simulink model "AirCtl_CtlValCalc"  (R2016b)
settings: configuration reference "CodeGenConfigSet" (kept outside this file)
values from neighbouring files (symbols this model uses):
  AirCtl_drCtlValDec_CUR = Calibration.Parameter    [init_AirCtl_CtlValCalc.m]    (also in init_AirCtl_CtlValCalc_SIL.m = Simulink.Parameter)
  AirCtl_drCtlValDec_CURX = Calibration.Parameter    [init_AirCtl_CtlValCalc.m]    (also in init_AirCtl_CtlValCalc_SIL.m = Simulink.Parameter)
  AirCtl_drCtlValDwn_C = Calibration.Parameter    [init_AirCtl_CtlValCalc.m]    (also in init_AirCtl_CtlValCalc_SIL.m = Simulink.Parameter)
  AirCtl_drCtlValInc_CUR = Calibration.Parameter    [init_AirCtl_CtlValCalc.m]    (also in init_AirCtl_CtlValCalc_SIL.m = Simulink.Parameter)
  AirCtl_drCtlValInc_CURX = Calibration.Parameter    [init_AirCtl_CtlValCalc.m]    (also in init_AirCtl_CtlValCalc_SIL.m = Simulink.Parameter)
  AirCtl_drCtlValUp_C = Calibration.Parameter    [init_AirCtl_CtlValCalc.m]    (also in init_AirCtl_CtlValCalc_SIL.m = Simulink.Parameter)
  AirCtl_facCtlAirTempCorEOM0_CUR = Calibration.Parameter    [init_AirCtl_CtlValCalc.m]    (also in init_AirCtl_CtlValCalc_SIL.m = Simulink.Parameter)
  AirCtl_facCtlAirTempCorEOM0_CURX = Calibration.Parameter    [init_AirCtl_CtlValCalc.m]    (also in init_AirCtl_CtlValCalc_SIL.m = Simulink.Parameter)
  AirCtl_facCtlEngTempCorEOM0_CUR = Calibration.Parameter    [init_AirCtl_CtlValCalc.m]    (also in init_AirCtl_CtlValCalc_SIL.m = Simulink.Parameter)
  AirCtl_facCtlEngTempCorEOM0_CURX = Calibration.Parameter    [init_AirCtl_CtlValCalc.m]    (also in init_AirCtl_CtlValCalc_SIL.m = Simulink.Parameter)
  AirCtl_facEngTempSmkDynCor_CUR = Calibration.Parameter    [init_AirCtl_CtlValCalc.m]    (also in init_AirCtl_CtlValCalc_SIL.m = Simulink.Parameter)
  AirCtl_facEngTempSmkDynCor_CURX = Calibration.Parameter    [init_AirCtl_CtlValCalc.m]    (also in init_AirCtl_CtlValCalc_SIL.m = Simulink.Parameter)
  AirCtl_facEngTempSmkStatCor_CUR = Calibration.Parameter    [init_AirCtl_CtlValCalc.m]    (also in init_AirCtl_CtlValCalc_SIL.m = Simulink.Parameter)
  AirCtl_facEngTempSmkStatCor_CURX = Calibration.Parameter    [init_AirCtl_CtlValCalc.m]    (also in init_AirCtl_CtlValCalc_SIL.m = Simulink.Parameter)
  AirCtl_facEnvPresCtlVal_CUR = Calibration.Parameter    [init_AirCtl_CtlValCalc.m]    (also in init_AirCtl_CtlValCalc_SIL.m = Simulink.Parameter)
  AirCtl_facEnvPresCtlVal_CURX = Calibration.Parameter    [init_AirCtl_CtlValCalc.m]    (also in init_AirCtl_CtlValCalc_SIL.m = Simulink.Parameter)
  AirCtl_facWrmUpCtlVal_CUR = Calibration.Parameter    [init_AirCtl_CtlValCalc.m]    (also in init_AirCtl_CtlValCalc_SIL.m = Simulink.Parameter)
  AirCtl_facWrmUpCtlVal_CURX = Calibration.Parameter    [init_AirCtl_CtlValCalc.m]    (also in init_AirCtl_CtlValCalc_SIL.m = Simulink.Parameter)
  AirCtl_numAirTempCtlVal_C = Calibration.Parameter    [init_AirCtl_CtlValCalc.m]    (also in init_AirCtl_CtlValCalc_SIL.m = Simulink.Parameter)
  AirCtl_numEngTempCtlVal_C = Calibration.Parameter    [init_AirCtl_CtlValCalc.m]    (also in init_AirCtl_CtlValCalc_SIL.m = Simulink.Parameter)
  AirCtl_rCtlAirTempCorEOM0_MAP = Calibration.Parameter    [init_AirCtl_CtlValCalc.m]    (also in init_AirCtl_CtlValCalc_SIL.m = Simulink.Parameter)
  AirCtl_rCtlAirTempCorEOM0_MAPX = Calibration.Parameter    [init_AirCtl_CtlValCalc.m]    (also in init_AirCtl_CtlValCalc_SIL.m = Simulink.Parameter)
  AirCtl_rCtlAirTempCorEOM0_MAPY = Calibration.Parameter    [init_AirCtl_CtlValCalc.m]    (also in init_AirCtl_CtlValCalc_SIL.m = Simulink.Parameter)
  AirCtl_rCtlCorBasEOM0_MAP = Calibration.Parameter    [init_AirCtl_CtlValCalc.m]    (also in init_AirCtl_CtlValCalc_SIL.m = Simulink.Parameter)
  AirCtl_rCtlCorBasEOM0_MAPX = Calibration.Parameter    [init_AirCtl_CtlValCalc.m]    (also in init_AirCtl_CtlValCalc_SIL.m = Simulink.Parameter)
  AirCtl_rCtlCorBasEOM0_MAPY = Calibration.Parameter    [init_AirCtl_CtlValCalc.m]    (also in init_AirCtl_CtlValCalc_SIL.m = Simulink.Parameter)
  AirCtl_rCtlEngTempCorEOM0_MAP = Calibration.Parameter    [init_AirCtl_CtlValCalc.m]    (also in init_AirCtl_CtlValCalc_SIL.m = Simulink.Parameter)
  AirCtl_rCtlEngTempCorEOM0_MAPX = Calibration.Parameter    [init_AirCtl_CtlValCalc.m]    (also in init_AirCtl_CtlValCalc_SIL.m = Simulink.Parameter)
  AirCtl_rCtlEngTempCorEOM0_MAPY = Calibration.Parameter    [init_AirCtl_CtlValCalc.m]    (also in init_AirCtl_CtlValCalc_SIL.m = Simulink.Parameter)
  AirCtl_rCtlEnvPresCorEOM0_MAP = Calibration.Parameter    [init_AirCtl_CtlValCalc.m]    (also in init_AirCtl_CtlValCalc_SIL.m = Simulink.Parameter)
  AirCtl_rCtlEnvPresCorEOM0_MAPX = Calibration.Parameter    [init_AirCtl_CtlValCalc.m]    (also in init_AirCtl_CtlValCalc_SIL.m = Simulink.Parameter)
  AirCtl_rCtlEnvPresCorEOM0_MAPY = Calibration.Parameter    [init_AirCtl_CtlValCalc.m]    (also in init_AirCtl_CtlValCalc_SIL.m = Simulink.Parameter)
  AirCtl_rCtlValBasEOM0_MAP = Calibration.Parameter    [init_AirCtl_CtlValCalc.m]    (also in init_AirCtl_CtlValCalc_SIL.m = Simulink.Parameter)
  AirCtl_rCtlValBasEOM0_MAPX = Calibration.Parameter    [init_AirCtl_CtlValCalc.m]    (also in init_AirCtl_CtlValCalc_SIL.m = Simulink.Parameter)
  AirCtl_rCtlValBasEOM0_MAPY = Calibration.Parameter    [init_AirCtl_CtlValCalc.m]    (also in init_AirCtl_CtlValCalc_SIL.m = Simulink.Parameter)
  AirCtl_rEngTempSmkDynCor_MAP = Calibration.Parameter    [init_AirCtl_CtlValCalc.m]    (also in init_AirCtl_CtlValCalc_SIL.m = Simulink.Parameter)
  AirCtl_rEngTempSmkDynCor_MAPX = Calibration.Parameter    [init_AirCtl_CtlValCalc.m]    (also in init_AirCtl_CtlValCalc_SIL.m = Simulink.Parameter)
  AirCtl_rEngTempSmkDynCor_MAPY = Calibration.Parameter    [init_AirCtl_CtlValCalc.m]    (also in init_AirCtl_CtlValCalc_SIL.m = Simulink.Parameter)
  AirCtl_rEngTempSmkStatCor_MAP = Calibration.Parameter    [init_AirCtl_CtlValCalc.m]    (also in init_AirCtl_CtlValCalc_SIL.m = Simulink.Parameter)
  AirCtl_rEngTempSmkStatCor_MAPX = Calibration.Parameter    [init_AirCtl_CtlValCalc.m]    (also in init_AirCtl_CtlValCalc_SIL.m = Simulink.Parameter)
  AirCtl_rEngTempSmkStatCor_MAPY = Calibration.Parameter    [init_AirCtl_CtlValCalc.m]    (also in init_AirCtl_CtlValCalc_SIL.m = Simulink.Parameter)
  AirCtl_rEnvPresCtlVal_MAP = Calibration.Parameter    [init_AirCtl_CtlValCalc.m]    (also in init_AirCtl_CtlValCalc_SIL.m = Simulink.Parameter)
  AirCtl_rEnvPresCtlVal_MAPX = Calibration.Parameter    [init_AirCtl_CtlValCalc.m]    (also in init_AirCtl_CtlValCalc_SIL.m = Simulink.Parameter)
  AirCtl_rEnvPresCtlVal_MAPY = Calibration.Parameter    [init_AirCtl_CtlValCalc.m]    (also in init_AirCtl_CtlValCalc_SIL.m = Simulink.Parameter)
  AirCtl_rSmkDyn_MAP = Calibration.Parameter    [init_AirCtl_CtlValCalc.m]    (also in init_AirCtl_CtlValCalc_SIL.m = Simulink.Parameter)
  AirCtl_rSmkDyn_MAPX = Calibration.Parameter    [init_AirCtl_CtlValCalc.m]    (also in init_AirCtl_CtlValCalc_SIL.m = Simulink.Parameter)
  AirCtl_rSmkDyn_MAPY = Calibration.Parameter    [init_AirCtl_CtlValCalc.m]    (also in init_AirCtl_CtlValCalc_SIL.m = Simulink.Parameter)
  AirCtl_rSmkStat_MAP = Calibration.Parameter    [init_AirCtl_CtlValCalc.m]    (also in init_AirCtl_CtlValCalc_SIL.m = Simulink.Parameter)
  AirCtl_rSmkStat_MAPX = Calibration.Parameter    [init_AirCtl_CtlValCalc.m]    (also in init_AirCtl_CtlValCalc_SIL.m = Simulink.Parameter)
  AirCtl_rSmkStat_MAPY = Calibration.Parameter    [init_AirCtl_CtlValCalc.m]    (also in init_AirCtl_CtlValCalc_SIL.m = Simulink.Parameter)
  AirCtl_rWrmUpCtlVal_MAP = Calibration.Parameter    [init_AirCtl_CtlValCalc.m]    (also in init_AirCtl_CtlValCalc_SIL.m = Simulink.Parameter)
  AirCtl_rWrmUpCtlVal_MAPX = Calibration.Parameter    [init_AirCtl_CtlValCalc.m]    (also in init_AirCtl_CtlValCalc_SIL.m = Simulink.Parameter)
  AirCtl_rWrmUpCtlVal_MAPY = Calibration.Parameter    [init_AirCtl_CtlValCalc.m]    (also in init_AirCtl_CtlValCalc_SIL.m = Simulink.Parameter)
  AirCtl_swtAirMs_C = Calibration.Parameter    [init_AirCtl_CtlValCalc.m]    (also in init_AirCtl_CtlValCalc_SIL.m = Simulink.Parameter)
undefined symbols (not defined in the file or in its folder): AirCtl_CtlValCalc_DT, Switch_conv
libraries: CXLib x6
settings Model: Creator=lvzhanghui  LastModifiedBy=zhulinfeng
settings ConfigSetRef: SourceLocation=Base Workspace

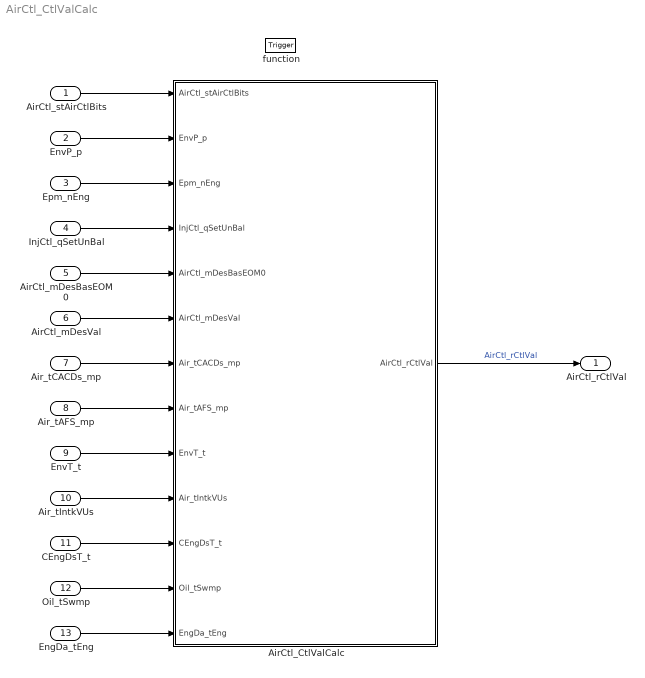
== system AirCtl_CtlValCalc ==
  AirCtl_stAirCtlBits : Inport  Description=Status of the switch-off events of the exhaust-gas recirculation control, monitoring  OutMin=0  OutMax=4294967295  OutDataTypeStr=State_uint32
  EnvP_p : Inport  Tag=kPa  Description=Barometric pressure  Port=2  OutMin=0  OutMax=3276  OutDataTypeStr=AirPressure_kPa
  Epm_nEng : Inport  Tag=rpm  Description=Engine speed  Port=3  OutMin=0  OutMax=6000  OutDataTypeStr=EngSpeed_rpm
  InjCtl_qSetUnBal : Inport  Tag=mg/hub  Description=Current injection quantity  Port=4  OutMin=-319  OutMax=319  OutDataTypeStr=FuelMass_mg_hub
  AirCtl_mDesBasEOM0 : Inport  Tag=mg/hub  Description=Base air mass setpoint value from the basic map  Port=5  OutMin=-15000  OutMax=15000  OutDataTypeStr=AirMass_mg_hub
  AirCtl_mDesVal : Inport  Tag=mg/hub  Description=Desired air mass  Port=6  OutMin=-15000  OutMax=15000  OutDataTypeStr=AirMass_mg_hub
  Air_tCACDs_mp : Inport  Tag=deg  Description=Charge-air temperature downstream from charge-air cooler  Port=7  OutMin=-200  OutMax=200  OutDataTypeStr=Temp_deg
  Air_tAFS_mp : Inport  Tag=deg  Description=Induction air temperature at the HFM  Port=8  OutMin=-200  OutMax=200  OutDataTypeStr=Temp_deg
  EnvT_t : Inport  Tag=deg  Description=Environmental temperature  Port=9  OutMin=-200  OutMax=200  OutDataTypeStr=Temp_deg
  Air_tIntkVUs : Inport  Tag=deg  Description=Intake air temperature upstream of the inlet valve  Port=10  OutMin=-200  OutMax=200  OutDataTypeStr=Temp_deg
  CEngDsT_t : Inport  Tag=deg  Description=engine coolant temperature after filter  Port=11  OutMin=-200  OutMax=200  OutDataTypeStr=Temp_deg
  Oil_tSwmp : Inport  Tag=deg  Description=Oil temperature in oil sump  Port=12  OutMin=-50  OutMax=200  OutDataTypeStr=Temp_deg
  EngDa_tEng : Inport  Tag=deg  Description=Engine temperature  Port=13  OutMin=-1000  OutMax=1000  OutDataTypeStr=Temp_deg
  function : TriggerPort  TriggerType=function-call  VariantControl=Variant
  AirCtl_CtlValCalc : Subsystem
  AirCtl_rCtlVal : Outport  Tag=%  Description=Stationary part of controlled variable  OutMin=-100  OutMax=100  OutDataTypeStr=Prc_100_rate
  wires:
  AirCtl_CtlValCalc/1(AirCtl_rCtlVal) -> AirCtl_rCtlVal/1  "AirCtl_rCtlVal"
  EngDa_tEng/1 -> AirCtl_CtlValCalc/13(EngDa_tEng)
  Oil_tSwmp/1 -> AirCtl_CtlValCalc/12(Oil_tSwmp)
  CEngDsT_t/1 -> AirCtl_CtlValCalc/11(CEngDsT_t)
  Air_tIntkVUs/1 -> AirCtl_CtlValCalc/10(Air_tIntkVUs)
  EnvT_t/1 -> AirCtl_CtlValCalc/9(EnvT_t)
  Air_tAFS_mp/1 -> AirCtl_CtlValCalc/8(Air_tAFS_mp)
  Air_tCACDs_mp/1 -> AirCtl_CtlValCalc/7(Air_tCACDs_mp)
  AirCtl_mDesVal/1 -> AirCtl_CtlValCalc/6(AirCtl_mDesVal)
  AirCtl_mDesBasEOM0/1 -> AirCtl_CtlValCalc/5(AirCtl_mDesBasEOM0)
  InjCtl_qSetUnBal/1 -> AirCtl_CtlValCalc/4(InjCtl_qSetUnBal)
  Epm_nEng/1 -> AirCtl_CtlValCalc/3(Epm_nEng)
  EnvP_p/1 -> AirCtl_CtlValCalc/2(EnvP_p)
  AirCtl_stAirCtlBits/1 -> AirCtl_CtlValCalc/1(AirCtl_stAirCtlBits)

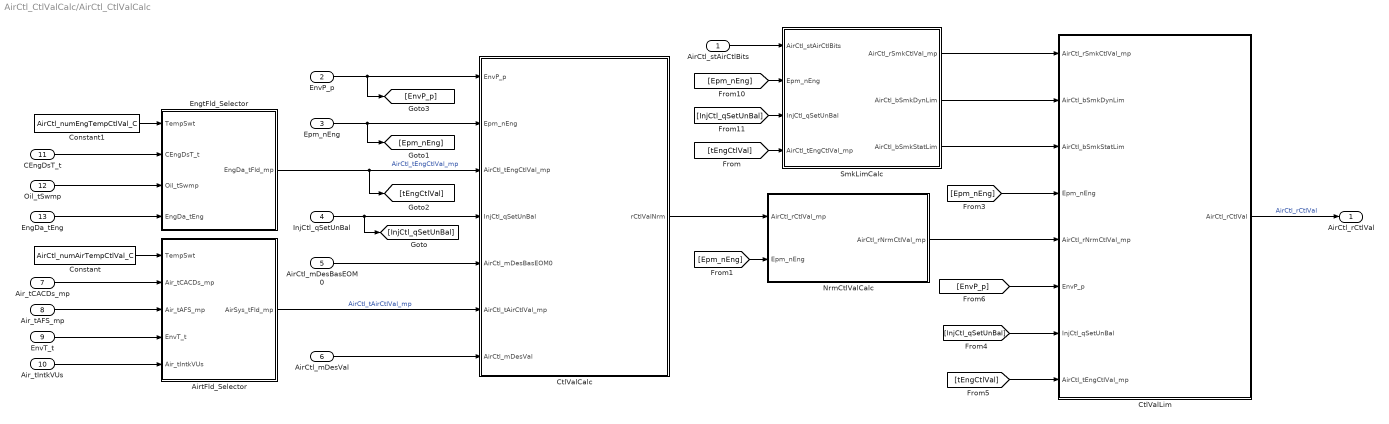
== system AirCtl_CtlValCalc/AirCtl_CtlValCalc ==
  AirCtl_stAirCtlBits : Inport
  EnvP_p : Inport  Tag=kPa  Port=2
  Epm_nEng : Inport  Tag=rpm  Port=3
  InjCtl_qSetUnBal : Inport  Tag=mg/hub  Port=4
  AirCtl_mDesBasEOM0 : Inport  Tag=mg/hub  Port=5
  AirCtl_mDesVal : Inport  Tag=mg/hub  Port=6
  Air_tCACDs_mp : Inport  Tag=deg  Port=7
  Air_tAFS_mp : Inport  Tag=deg  Port=8
  EnvT_t : Inport  Tag=deg  Port=9
  Air_tIntkVUs : Inport  Tag=deg  Port=10
  CEngDsT_t : Inport  Tag=deg  Port=11
  Oil_tSwmp : Inport  Tag=deg  Port=12
  EngDa_tEng : Inport  Tag=deg  Port=13
  AirtFld_Selector : Subsystem
  Constant : Constant  Value=AirCtl_numAirTempCtlVal_C
  Constant1 : Constant  Value=AirCtl_numEngTempCtlVal_C
  CtlValCalc : Subsystem
  CtlValLim : Subsystem
  EngtFld_Selector : Subsystem
  NrmCtlValCalc : Subsystem
  SmkLimCalc : Subsystem
  AirCtl_rCtlVal : Outport  Tag=%
  wires:
  SmkLimCalc/2(AirCtl_bSmkDynLim) -> CtlValLim/2(AirCtl_bSmkDynLim)
  Constant/1 -> AirtFld_Selector/1(TempSwt)
  NrmCtlValCalc/1(AirCtl_rNrmCtlVal_mp) -> CtlValLim/5(AirCtl_rNrmCtlVal_mp)
  EngtFld_Selector/1(EngDa_tFld_mp) -> [tEngCtlVal], CtlValCalc/3(AirCtl_tEngCtlVal_mp)  "AirCtl_tEngCtlVal_mp"
  SmkLimCalc/3(AirCtl_bSmkStatLim) -> CtlValLim/3(AirCtl_bSmkStatLim)
  AirtFld_Selector/1(AirSys_tFld_mp) -> CtlValCalc/6(AirCtl_tAirCtlVal_mp)  "AirCtl_tAirCtlVal_mp"
  Epm_nEng/1 -> [Epm_nEng], CtlValCalc/2(Epm_nEng)
  Constant1/1 -> EngtFld_Selector/1(TempSwt)
  InjCtl_qSetUnBal/1 -> [InjCtl_qSetUnBal], CtlValCalc/4(InjCtl_qSetUnBal)
  EnvP_p/1 -> CtlValCalc/1(EnvP_p), [EnvP_p]
  SmkLimCalc/1(AirCtl_rSmkCtlVal_mp) -> CtlValLim/1(AirCtl_rSmkCtlVal_mp)
  Air_tCACDs_mp/1 -> AirtFld_Selector/2(Air_tCACDs_mp)
  Air_tAFS_mp/1 -> AirtFld_Selector/3(Air_tAFS_mp)
  EnvT_t/1 -> AirtFld_Selector/4(EnvT_t)
  Air_tIntkVUs/1 -> AirtFld_Selector/5(Air_tIntkVUs)
  AirCtl_mDesVal/1 -> CtlValCalc/7(AirCtl_mDesVal)
  [Epm_nEng] -> CtlValLim/4(Epm_nEng)
  [EnvP_p] -> CtlValLim/6(EnvP_p)
  [InjCtl_qSetUnBal] -> CtlValLim/7(InjCtl_qSetUnBal)
  [tEngCtlVal] -> CtlValLim/8(AirCtl_tEngCtlVal_mp)
  CEngDsT_t/1 -> EngtFld_Selector/2(CEngDsT_t)
  Oil_tSwmp/1 -> EngtFld_Selector/3(Oil_tSwmp)
  EngDa_tEng/1 -> EngtFld_Selector/4(EngDa_tEng)
  [Epm_nEng] -> NrmCtlValCalc/2(Epm_nEng)
  [Epm_nEng] -> SmkLimCalc/2(Epm_nEng)
  [InjCtl_qSetUnBal] -> SmkLimCalc/3(InjCtl_qSetUnBal)
  AirCtl_stAirCtlBits/1 -> SmkLimCalc/1(AirCtl_stAirCtlBits)
  [tEngCtlVal] -> SmkLimCalc/4(AirCtl_tEngCtlVal_mp)
  CtlValLim/1(AirCtl_rCtlVal) -> AirCtl_rCtlVal/1  "AirCtl_rCtlVal"
  CtlValCalc/1(rCtlValNrm) -> NrmCtlValCalc/1(AirCtl_rCtlVal_mp)
  AirCtl_mDesBasEOM0/1 -> CtlValCalc/5(AirCtl_mDesBasEOM0)

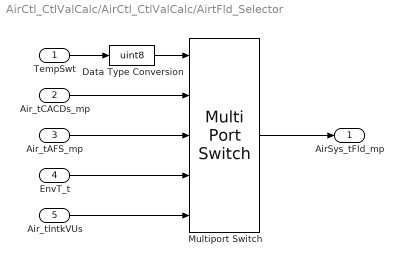
== system AirCtl_CtlValCalc/AirCtl_CtlValCalc/AirtFld_Selector ==
  TempSwt : Inport
  Air_tCACDs_mp : Inport  Tag=deg  Port=2
  Air_tAFS_mp : Inport  Tag=deg  Port=3
  EnvT_t : Inport  Tag=deg  Port=4
  Air_tIntkVUs : Inport  Tag=deg  Port=5
  Data Type Conversion : DataTypeConversion  OutDataTypeStr=uint8
  Multiport Switch : MultiPortSwitch  DataPortOrder=Zero-based contiguous  Inputs=4
  AirSys_tFld_mp : Outport  Tag=deg
  wires:
  Air_tCACDs_mp/1 -> Multiport Switch/2
  Multiport Switch/1 -> AirSys_tFld_mp/1
  EnvT_t/1 -> Multiport Switch/4
  Air_tAFS_mp/1 -> Multiport Switch/3
  Data Type Conversion/1 -> Multiport Switch/1
  TempSwt/1 -> Data Type Conversion/1
  Air_tIntkVUs/1 -> Multiport Switch/5

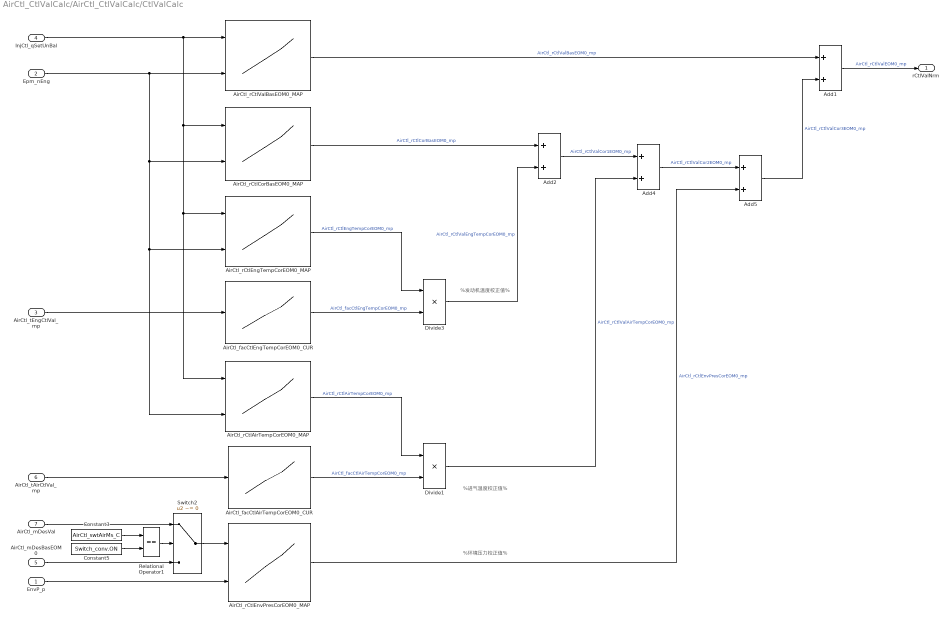
== system AirCtl_CtlValCalc/AirCtl_CtlValCalc/CtlValCalc ==
  note: %环境压力校正值%
  note: %发动机温度校正值%
  note: %进气温度校正值%
  EnvP_p : Inport
  Epm_nEng : Inport  Port=2
  AirCtl_tEngCtlVal_mp : Inport  Port=3
  InjCtl_qSetUnBal : Inport  Port=4
  AirCtl_mDesBasEOM0 : Inport  Port=5
  AirCtl_tAirCtlVal_mp : Inport  Port=6
  AirCtl_mDesVal : Inport  Port=7
  Add{1..2,4..5} (4 alike) : Sum  SaturateOnIntegerOverflow=on  InputSameDT=on
  AirCtl_facCtlAirTempCorEOM0_CUR : Lookup_n-D  NumberOfTableDimensions=1  BreakpointsForDimension1=AirCtl_facCtlAirTempCorEOM0_CURX  BeginIndexSearchUsingPreviousIndexResult=on  Table=AirCtl_facCtlAirTempCorEOM0_CUR  TableDataTypeStr=Inherit: Inherit from 'Table data'  ExtrapMethod=Clip  UseLastTableValue=on  InternalRulePriority=Speed  OutDataTypeStr=Inherit: Inherit from 'Table data'  RndMeth=Simplest  SaturateOnIntegerOverflow=on
  AirCtl_facCtlEngTempCorEOM0_CUR : Lookup_n-D  NumberOfTableDimensions=1  BreakpointsForDimension1=AirCtl_facCtlEngTempCorEOM0_CURX  BeginIndexSearchUsingPreviousIndexResult=on  Table=AirCtl_facCtlEngTempCorEOM0_CUR  TableDataTypeStr=Inherit: Inherit from 'Table data'  ExtrapMethod=Clip  UseLastTableValue=on  InternalRulePriority=Speed  OutDataTypeStr=Inherit: Inherit from 'Table data'  RndMeth=Simplest  SaturateOnIntegerOverflow=on
  AirCtl_rCtlAirTempCorEOM0_MAP : Lookup_n-D  BreakpointsForDimension1=AirCtl_rCtlAirTempCorEOM0_MAPY  BreakpointsForDimension2=AirCtl_rCtlAirTempCorEOM0_MAPX  BeginIndexSearchUsingPreviousIndexResult=on  Table=AirCtl_rCtlAirTempCorEOM0_MAP  TableDataTypeStr=Inherit: Inherit from 'Table data'  ExtrapMethod=Clip  UseLastTableValue=on  InternalRulePriority=Speed  OutDataTypeStr=Inherit: Inherit from 'Table data'  RndMeth=Simplest  SaturateOnIntegerOverflow=on
  AirCtl_rCtlCorBasEOM0_MAP : Lookup_n-D  BreakpointsForDimension1=AirCtl_rCtlCorBasEOM0_MAPY  BreakpointsForDimension2=AirCtl_rCtlCorBasEOM0_MAPX  BeginIndexSearchUsingPreviousIndexResult=on  Table=AirCtl_rCtlCorBasEOM0_MAP  TableDataTypeStr=Inherit: Inherit from 'Table data'  ExtrapMethod=Clip  UseLastTableValue=on  InternalRulePriority=Speed  OutDataTypeStr=Inherit: Inherit from 'Table data'  RndMeth=Simplest  SaturateOnIntegerOverflow=on
  AirCtl_rCtlEngTempCorEOM0_MAP : Lookup_n-D  BreakpointsForDimension1=AirCtl_rCtlEngTempCorEOM0_MAPY  BreakpointsForDimension2=AirCtl_rCtlEngTempCorEOM0_MAPX  BeginIndexSearchUsingPreviousIndexResult=on  Table=AirCtl_rCtlEngTempCorEOM0_MAP  TableDataTypeStr=Inherit: Inherit from 'Table data'  ExtrapMethod=Clip  UseLastTableValue=on  InternalRulePriority=Speed  OutDataTypeStr=Inherit: Inherit from 'Table data'  RndMeth=Simplest  SaturateOnIntegerOverflow=on
  AirCtl_rCtlEnvPresCorEOM0_MAP : Lookup_n-D  BreakpointsForDimension1=AirCtl_rCtlEnvPresCorEOM0_MAPY  BreakpointsForDimension2=AirCtl_rCtlEnvPresCorEOM0_MAPX  BeginIndexSearchUsingPreviousIndexResult=on  Table=AirCtl_rCtlEnvPresCorEOM0_MAP  TableDataTypeStr=Inherit: Inherit from 'Table data'  ExtrapMethod=Clip  UseLastTableValue=on  InternalRulePriority=Speed  OutDataTypeStr=Inherit: Inherit from 'Table data'  RndMeth=Simplest  SaturateOnIntegerOverflow=on
  AirCtl_rCtlValBasEOM0_MAP : Lookup_n-D  BreakpointsForDimension1=AirCtl_rCtlValBasEOM0_MAPY  BreakpointsForDimension2=AirCtl_rCtlValBasEOM0_MAPX  BeginIndexSearchUsingPreviousIndexResult=on  Table=AirCtl_rCtlValBasEOM0_MAP  TableDataTypeStr=Inherit: Inherit from 'Table data'  ExtrapMethod=Clip  UseLastTableValue=on  InternalRulePriority=Speed  OutDataTypeStr=Inherit: Inherit from 'Table data'  RndMeth=Simplest  SaturateOnIntegerOverflow=on
  Constant3 : Constant  Value=AirCtl_swtAirMs_C
  Constant5 : Constant  Value=Switch_conv.ON
  Divide1 : Product  Inputs=**  OutDataTypeStr=Inherit: Inherit via back propagation  SaturateOnIntegerOverflow=on
  Divide3 : Product  Inputs=**  OutDataTypeStr=Inherit: Inherit via back propagation  SaturateOnIntegerOverflow=on
  Relational Operator1 : RelationalOperator  Operator===  OutDataTypeStr=boolean  RndMeth=Simplest  InputSameDT=on
  Switch2 : Switch  Criteria=u2 ~= 0  InputSameDT=on
  rCtlValNrm : Outport
  wires:
  Relational Operator1/1 -> Switch2/2
  Constant5/1 -> Relational Operator1/2
  Add5/1 -> Add1/2  "AirCtl_rCtlValCor3EOM0_mp"
  AirCtl_rCtlEnvPresCorEOM0_MAP/1 -> Add5/2  "AirCtl_rCtlEnvPresCorEOM0_mp"
  Add4/1 -> Add5/1  "AirCtl_rCtlValCor2EOM0_mp"
  Divide1/1 -> Add4/2  "AirCtl_rCtlValAirTempCorEOM0_mp"
  AirCtl_facCtlAirTempCorEOM0_CUR/1 -> Divide1/2  "AirCtl_facCtlAirTempCorEOM0_mp"
  AirCtl_rCtlAirTempCorEOM0_MAP/1 -> Divide1/1  "AirCtl_rCtlAirTempCorEOM0_mp"
  Divide3/1 -> Add2/2  "AirCtl_rCtlValEngTempCorEOM0_mp"
  AirCtl_facCtlEngTempCorEOM0_CUR/1 -> Divide3/2  "AirCtl_facCtlEngTempCorEOM0_mp"
  AirCtl_rCtlEngTempCorEOM0_MAP/1 -> Divide3/1  "AirCtl_rCtlEngTempCorEOM0_mp"
  Switch2/1 -> AirCtl_rCtlEnvPresCorEOM0_MAP/1
  Constant3/1 -> Relational Operator1/1
  Add1/1 -> rCtlValNrm/1  "AirCtl_rCtlValEOM0_mp"
  AirCtl_rCtlValBasEOM0_MAP/1 -> Add1/1  "AirCtl_rCtlValBasEOM0_mp"
  AirCtl_rCtlCorBasEOM0_MAP/1 -> Add2/1  "AirCtl_rCtlCorBasEOM0_mp"
  Add2/1 -> Add4/1  "AirCtl_rCtlValCor1EOM0_mp"
  EnvP_p/1 -> AirCtl_rCtlEnvPresCorEOM0_MAP/2
  AirCtl_tEngCtlVal_mp/1 -> AirCtl_facCtlEngTempCorEOM0_CUR/1
  AirCtl_tAirCtlVal_mp/1 -> AirCtl_facCtlAirTempCorEOM0_CUR/1
  AirCtl_mDesVal/1 -> Switch2/1
  Epm_nEng/1 -> AirCtl_rCtlValBasEOM0_MAP/2, AirCtl_rCtlCorBasEOM0_MAP/2, AirCtl_rCtlEngTempCorEOM0_MAP/2, AirCtl_rCtlAirTempCorEOM0_MAP/2
  AirCtl_mDesBasEOM0/1 -> Switch2/3
  InjCtl_qSetUnBal/1 -> AirCtl_rCtlValBasEOM0_MAP/1, AirCtl_rCtlCorBasEOM0_MAP/1, AirCtl_rCtlEngTempCorEOM0_MAP/1, AirCtl_rCtlAirTempCorEOM0_MAP/1

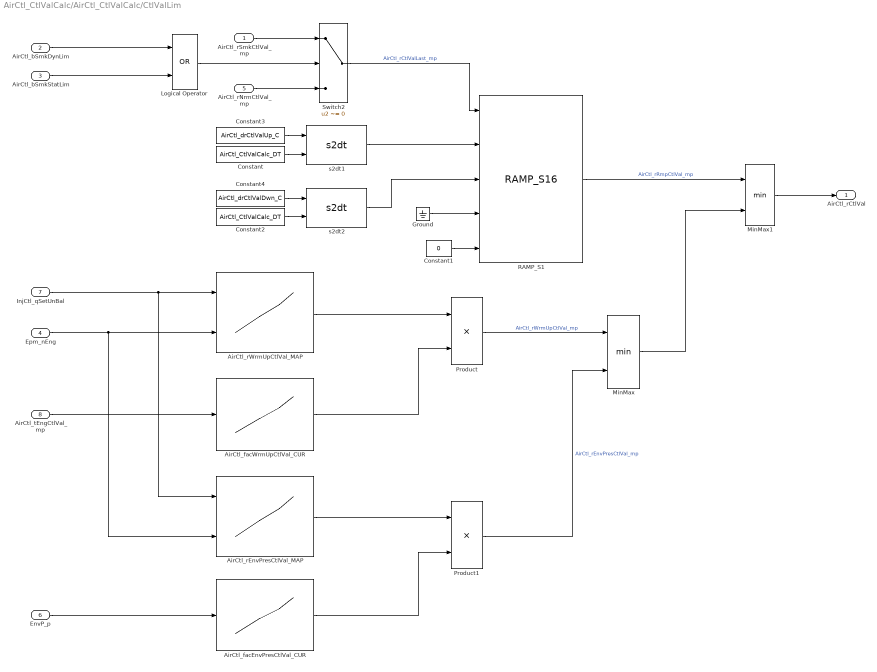
== system AirCtl_CtlValCalc/AirCtl_CtlValCalc/CtlValLim ==
  AirCtl_rSmkCtlVal_mp : Inport
  AirCtl_bSmkDynLim : Inport  Port=2
  AirCtl_bSmkStatLim : Inport  Port=3
  Epm_nEng : Inport  Port=4
  AirCtl_rNrmCtlVal_mp : Inport  Port=5
  EnvP_p : Inport  Port=6
  InjCtl_qSetUnBal : Inport  Port=7
  AirCtl_tEngCtlVal_mp : Inport  Port=8
  AirCtl_facEnvPresCtlVal_CUR : Lookup_n-D  NumberOfTableDimensions=1  BreakpointsForDimension1=AirCtl_facEnvPresCtlVal_CURX  BeginIndexSearchUsingPreviousIndexResult=on  Table=AirCtl_facEnvPresCtlVal_CUR  TableDataTypeStr=Inherit: Inherit from 'Table data'  ExtrapMethod=Clip  UseLastTableValue=on  InternalRulePriority=Speed  OutDataTypeStr=Inherit: Inherit from 'Table data'  RndMeth=Simplest  SaturateOnIntegerOverflow=on
  AirCtl_facWrmUpCtlVal_CUR : Lookup_n-D  NumberOfTableDimensions=1  BreakpointsForDimension1=AirCtl_facWrmUpCtlVal_CURX  BeginIndexSearchUsingPreviousIndexResult=on  Table=AirCtl_facWrmUpCtlVal_CUR  TableDataTypeStr=Inherit: Inherit from 'Table data'  ExtrapMethod=Clip  UseLastTableValue=on  InternalRulePriority=Speed  OutDataTypeStr=Inherit: Inherit from 'Table data'  RndMeth=Simplest  SaturateOnIntegerOverflow=on
  AirCtl_rEnvPresCtlVal_MAP : Lookup_n-D  BreakpointsForDimension1=AirCtl_rEnvPresCtlVal_MAPY  BreakpointsForDimension2=AirCtl_rEnvPresCtlVal_MAPX  BeginIndexSearchUsingPreviousIndexResult=on  Table=AirCtl_rEnvPresCtlVal_MAP  TableDataTypeStr=Inherit: Inherit from 'Table data'  ExtrapMethod=Clip  UseLastTableValue=on  InternalRulePriority=Speed  OutDataTypeStr=Inherit: Inherit from 'Table data'  RndMeth=Simplest  SaturateOnIntegerOverflow=on
  AirCtl_rWrmUpCtlVal_MAP : Lookup_n-D  BreakpointsForDimension1=AirCtl_rWrmUpCtlVal_MAPY  BreakpointsForDimension2=AirCtl_rWrmUpCtlVal_MAPX  BeginIndexSearchUsingPreviousIndexResult=on  Table=AirCtl_rWrmUpCtlVal_MAP  TableDataTypeStr=Inherit: Inherit from 'Table data'  ExtrapMethod=Clip  UseLastTableValue=on  InternalRulePriority=Speed  OutDataTypeStr=Inherit: Inherit from 'Table data'  RndMeth=Simplest  SaturateOnIntegerOverflow=on
  Constant : Constant  Value=AirCtl_CtlValCalc_DT
  Constant1 : Constant  Value=0  OutDataTypeStr=Inherit: Inherit via back propagation
  Constant2 : Constant  Value=AirCtl_CtlValCalc_DT
  Constant3 : Constant  Value=AirCtl_drCtlValUp_C
  Constant4 : Constant  Value=AirCtl_drCtlValDwn_C
  Ground : Ground
  Logical Operator : Logic  Operator=OR  OutDataTypeStr=boolean
  MinMax : MinMax  Inputs=2
  MinMax1 : MinMax  Inputs=2
  Product : Product  OutDataTypeStr=Inherit: Inherit via back propagation  SaturateOnIntegerOverflow=on
  Product1 : Product  OutDataTypeStr=Inherit: Inherit via back propagation  SaturateOnIntegerOverflow=on
  RAMP_S1 : CXLib/RAMP_S16
  Switch2 : Switch  Criteria=u2 ~= 0  InputSameDT=on
  s2dt1 : CXLib/s2dt
  s2dt2 : CXLib/s2dt
  AirCtl_rCtlVal : Outport
  wires:
  s2dt2/1 -> RAMP_S1/3
  Constant2/1 -> s2dt2/2
  s2dt1/1 -> RAMP_S1/2
  Constant/1 -> s2dt1/2
  Ground/1 -> RAMP_S1/4
  Constant1/1 -> RAMP_S1/5
  AirCtl_bSmkStatLim/1 -> Logical Operator/2
  AirCtl_bSmkDynLim/1 -> Logical Operator/1
  Logical Operator/1 -> Switch2/2
  AirCtl_rNrmCtlVal_mp/1 -> Switch2/3
  AirCtl_rSmkCtlVal_mp/1 -> Switch2/1
  Switch2/1 -> RAMP_S1/1  "AirCtl_rCtlValLast_mp"
  Constant3/1 -> s2dt1/1
  Constant4/1 -> s2dt2/1
  Epm_nEng/1 -> AirCtl_rEnvPresCtlVal_MAP/2, AirCtl_rWrmUpCtlVal_MAP/2
  AirCtl_tEngCtlVal_mp/1 -> AirCtl_facWrmUpCtlVal_CUR/1
  EnvP_p/1 -> AirCtl_facEnvPresCtlVal_CUR/1
  InjCtl_qSetUnBal/1 -> AirCtl_rEnvPresCtlVal_MAP/1, AirCtl_rWrmUpCtlVal_MAP/1
  AirCtl_rWrmUpCtlVal_MAP/1 -> Product/1
  AirCtl_facWrmUpCtlVal_CUR/1 -> Product/2
  AirCtl_rEnvPresCtlVal_MAP/1 -> Product1/1
  AirCtl_facEnvPresCtlVal_CUR/1 -> Product1/2
  Product/1 -> MinMax/1  "AirCtl_rWrmUpCtlVal_mp"
  Product1/1 -> MinMax/2  "AirCtl_rEnvPresCtlVal_mp"
  RAMP_S1/1 -> MinMax1/1  "AirCtl_rRmpCtlVal_mp"
  MinMax/1 -> MinMax1/2
  MinMax1/1 -> AirCtl_rCtlVal/1

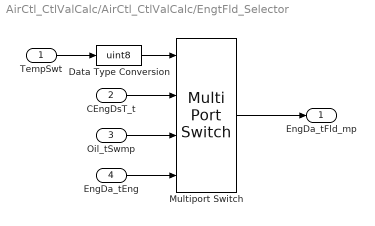
== system AirCtl_CtlValCalc/AirCtl_CtlValCalc/EngtFld_Selector ==
  TempSwt : Inport
  CEngDsT_t : Inport  Tag=deg  Port=2
  Oil_tSwmp : Inport  Tag=deg  Port=3
  EngDa_tEng : Inport  Tag=deg  Port=4
  Data Type Conversion : DataTypeConversion  OutDataTypeStr=uint8
  Multiport Switch : MultiPortSwitch  DataPortOrder=Zero-based contiguous
  EngDa_tFld_mp : Outport  Tag=deg
  wires:
  CEngDsT_t/1 -> Multiport Switch/2
  Multiport Switch/1 -> EngDa_tFld_mp/1
  EngDa_tEng/1 -> Multiport Switch/4
  Oil_tSwmp/1 -> Multiport Switch/3
  Data Type Conversion/1 -> Multiport Switch/1
  TempSwt/1 -> Data Type Conversion/1

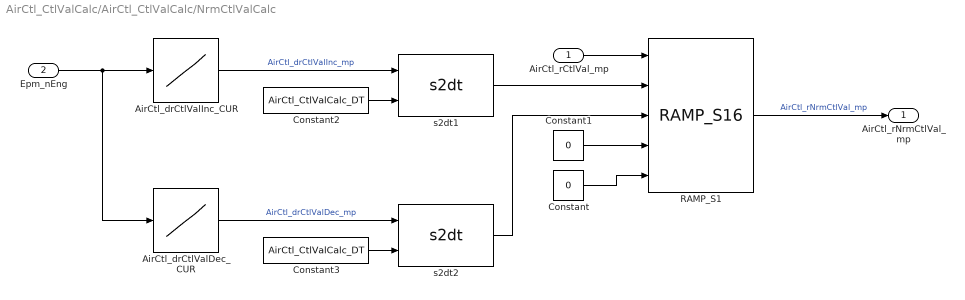
== system AirCtl_CtlValCalc/AirCtl_CtlValCalc/NrmCtlValCalc ==
  AirCtl_rCtlVal_mp : Inport
  Epm_nEng : Inport  Port=2
  AirCtl_drCtlValDec_CUR : Lookup_n-D  NumberOfTableDimensions=1  BreakpointsForDimension1=AirCtl_drCtlValDec_CURX  BeginIndexSearchUsingPreviousIndexResult=on  Table=AirCtl_drCtlValDec_CUR  TableDataTypeStr=Inherit: Inherit from 'Table data'  ExtrapMethod=Clip  UseLastTableValue=on  InternalRulePriority=Speed  OutDataTypeStr=Inherit: Inherit from 'Table data'  RndMeth=Simplest  SaturateOnIntegerOverflow=on
  AirCtl_drCtlValInc_CUR : Lookup_n-D  NumberOfTableDimensions=1  BreakpointsForDimension1=AirCtl_drCtlValInc_CURX  BeginIndexSearchUsingPreviousIndexResult=on  Table=AirCtl_drCtlValInc_CUR  TableDataTypeStr=Inherit: Inherit from 'Table data'  ExtrapMethod=Clip  UseLastTableValue=on  InternalRulePriority=Speed  OutDataTypeStr=Inherit: Inherit from 'Table data'  RndMeth=Simplest  SaturateOnIntegerOverflow=on
  Constant : Constant  Value=0  OutDataTypeStr=Inherit: Inherit via back propagation
  Constant1 : Constant  Value=0  OutDataTypeStr=Inherit: Inherit via back propagation
  Constant2 : Constant  Value=AirCtl_CtlValCalc_DT  OutDataTypeStr=Inherit: Inherit via back propagation
  Constant3 : Constant  Value=AirCtl_CtlValCalc_DT  OutDataTypeStr=Inherit: Inherit via back propagation
  RAMP_S1 : CXLib/RAMP_S16
  s2dt1 : CXLib/s2dt
  s2dt2 : CXLib/s2dt
  AirCtl_rNrmCtlVal_mp : Outport
  wires:
  Epm_nEng/1 -> AirCtl_drCtlValInc_CUR/1, AirCtl_drCtlValDec_CUR/1
  AirCtl_drCtlValInc_CUR/1 -> s2dt1/1  "AirCtl_drCtlValInc_mp"
  s2dt1/1 -> RAMP_S1/2
  AirCtl_drCtlValDec_CUR/1 -> s2dt2/1  "AirCtl_drCtlValDec_mp"
  s2dt2/1 -> RAMP_S1/3
  Constant1/1 -> RAMP_S1/4
  Constant/1 -> RAMP_S1/5
  Constant2/1 -> s2dt1/2
  Constant3/1 -> s2dt2/2
  AirCtl_rCtlVal_mp/1 -> RAMP_S1/1
  RAMP_S1/1 -> AirCtl_rNrmCtlVal_mp/1  "AirCtl_rNrmCtlVal_mp"

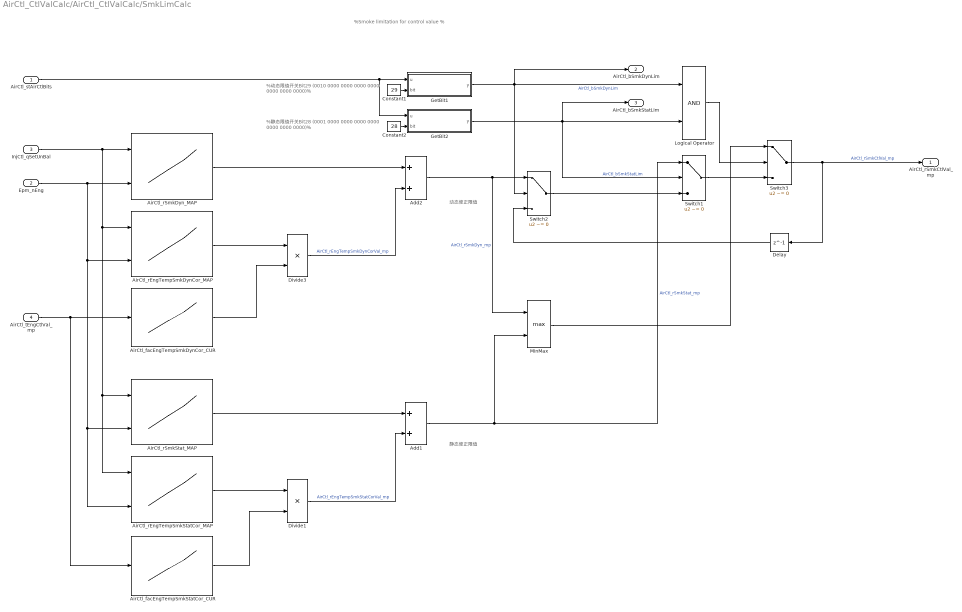
== system AirCtl_CtlValCalc/AirCtl_CtlValCalc/SmkLimCalc ==
  note: 静态修正限值
  note: 动态修正限值
  note: %Smoke limitation for control value %
  note: %动态限值开关Bit29
      | (0010 0000 0000 0000 0000 0000 0000 0000)%
  note: %静态限值开关Bit28
      | (0001 0000 0000 0000 0000 0000 0000 0000)%
  AirCtl_stAirCtlBits : Inport
  Epm_nEng : Inport  Port=2
  InjCtl_qSetUnBal : Inport  Port=3
  AirCtl_tEngCtlVal_mp : Inport  Port=4
  Add1 : Sum  SaturateOnIntegerOverflow=on  InputSameDT=on
  Add2 : Sum  SaturateOnIntegerOverflow=on  InputSameDT=on
  AirCtl_facEngTempSmkDynCor_CUR : Lookup_n-D  NumberOfTableDimensions=1  BreakpointsForDimension1=AirCtl_facEngTempSmkDynCor_CURX  BeginIndexSearchUsingPreviousIndexResult=on  Table=AirCtl_facEngTempSmkDynCor_CUR  TableDataTypeStr=Inherit: Inherit from 'Table data'  ExtrapMethod=Clip  UseLastTableValue=on  InternalRulePriority=Speed  OutDataTypeStr=Inherit: Inherit from 'Table data'  RndMeth=Simplest  SaturateOnIntegerOverflow=on
  AirCtl_facEngTempSmkStatCor_CUR : Lookup_n-D  NumberOfTableDimensions=1  BreakpointsForDimension1=AirCtl_facEngTempSmkStatCor_CURX  BeginIndexSearchUsingPreviousIndexResult=on  Table=AirCtl_facEngTempSmkStatCor_CUR  TableDataTypeStr=Inherit: Inherit from 'Table data'  ExtrapMethod=Clip  UseLastTableValue=on  InternalRulePriority=Speed  OutDataTypeStr=Inherit: Inherit from 'Table data'  RndMeth=Simplest  SaturateOnIntegerOverflow=on
  AirCtl_rEngTempSmkDynCor_MAP : Lookup_n-D  BreakpointsForDimension1=AirCtl_rEngTempSmkDynCor_MAPY  BreakpointsForDimension2=AirCtl_rEngTempSmkDynCor_MAPX  BeginIndexSearchUsingPreviousIndexResult=on  Table=AirCtl_rEngTempSmkDynCor_MAP  TableDataTypeStr=Inherit: Inherit from 'Table data'  ExtrapMethod=Clip  UseLastTableValue=on  InternalRulePriority=Speed  OutDataTypeStr=Inherit: Inherit from 'Table data'  RndMeth=Simplest  SaturateOnIntegerOverflow=on
  AirCtl_rEngTempSmkStatCor_MAP : Lookup_n-D  BreakpointsForDimension1=AirCtl_rEngTempSmkStatCor_MAPY  BreakpointsForDimension2=AirCtl_rEngTempSmkStatCor_MAPX  BeginIndexSearchUsingPreviousIndexResult=on  Table=AirCtl_rEngTempSmkStatCor_MAP  TableDataTypeStr=Inherit: Inherit from 'Table data'  ExtrapMethod=Clip  UseLastTableValue=on  InternalRulePriority=Speed  OutDataTypeStr=Inherit: Inherit from 'Table data'  RndMeth=Simplest  SaturateOnIntegerOverflow=on
  AirCtl_rSmkDyn_MAP : Lookup_n-D  BreakpointsForDimension1=AirCtl_rSmkDyn_MAPY  BreakpointsForDimension2=AirCtl_rSmkDyn_MAPX  BeginIndexSearchUsingPreviousIndexResult=on  Table=AirCtl_rSmkDyn_MAP  TableDataTypeStr=Inherit: Inherit from 'Table data'  ExtrapMethod=Clip  UseLastTableValue=on  InternalRulePriority=Speed  OutDataTypeStr=Inherit: Inherit from 'Table data'  RndMeth=Simplest  SaturateOnIntegerOverflow=on
  AirCtl_rSmkStat_MAP : Lookup_n-D  BreakpointsForDimension1=AirCtl_rSmkStat_MAPY  BreakpointsForDimension2=AirCtl_rSmkStat_MAPX  BeginIndexSearchUsingPreviousIndexResult=on  Table=AirCtl_rSmkStat_MAP  TableDataTypeStr=Inherit: Inherit from 'Table data'  ExtrapMethod=Clip  UseLastTableValue=on  InternalRulePriority=Speed  OutDataTypeStr=Inherit: Inherit from 'Table data'  RndMeth=Simplest  SaturateOnIntegerOverflow=on
  Constant1 : Constant  Value=29  OutDataTypeStr=uint8
  Constant2 : Constant  Value=28  OutDataTypeStr=uint8
  Delay : Delay  DelayLength=1  InitialCondition=0
  Divide1 : Product  Inputs=**  OutDataTypeStr=Inherit: Inherit via back propagation  SaturateOnIntegerOverflow=on
  Divide3 : Product  Inputs=**  OutDataTypeStr=Inherit: Inherit via back propagation  SaturateOnIntegerOverflow=on
  GetBit1 : Subsystem  mask(GetBit){dataTypeString=uint32, dataLength=0}
      mask prompts: dataTypeString "Input Data Type"; dataLength "DataType Length"
      mask help:
      | Acquires the value of the bit specified by the position (zero indexed).
      |
      | Output is always boolean.
      |
      | INPUTS:
      | u - input value
      | bit - position of bit to get (uint8)
      |
      | OUTPUTS:
      | y - output value
      mask init:
      | %Initial data type length info.
      | switch dataTypeString
      |     case 'uint8'
      |         dataLength=8;
      |     case 'uint16'
      |         dataLength=16;
      |     case 'uint32'
      |         dataLength=32;
      |     otherwise
      |         error('Unexpected data type define!')
      | end
      | set_param([get(gcbh,'path'),'/GetBit1/u'],'OutDataTypeStr',dataTypeString)
      settings: AttributesFormatString=Get bit from %<dataTypeString>
      mask Display: image(imread('GETBIT.jpg'),[0.2,0.2,0.6,0.6]);
  GetBit2 : Subsystem  mask(GetBit){dataTypeString=uint32, dataLength=0}
      mask prompts: dataTypeString "Input Data Type"; dataLength "DataType Length"
      mask help:
      | Acquires the value of the bit specified by the position (zero indexed).
      |
      | Output is always boolean.
      |
      | INPUTS:
      | u - input value
      | bit - position of bit to get (uint8)
      |
      | OUTPUTS:
      | y - output value
      mask init:
      | %Initial data type length info.
      | switch dataTypeString
      |     case 'uint8'
      |         dataLength=8;
      |     case 'uint16'
      |         dataLength=16;
      |     case 'uint32'
      |         dataLength=32;
      |     otherwise
      |         error('Unexpected data type define!')
      | end
      | set_param([get(gcbh,'path'),'/GetBit2/u'],'OutDataTypeStr',dataTypeString)
      settings: AttributesFormatString=Get bit from %<dataTypeString>
      mask Display: image(imread('GETBIT.jpg'),[0.2,0.2,0.6,0.6]);
  Logical Operator : Logic  OutDataTypeStr=boolean
  MinMax : MinMax  Function=max  Inputs=2  SaturateOnIntegerOverflow=on  InputSameDT=on
  Switch1 : Switch  Criteria=u2 ~= 0  SaturateOnIntegerOverflow=on  InputSameDT=on
  Switch2 : Switch  Criteria=u2 ~= 0  SaturateOnIntegerOverflow=on  InputSameDT=on
  Switch3 : Switch  Criteria=u2 ~= 0  SaturateOnIntegerOverflow=on  InputSameDT=on
  AirCtl_rSmkCtlVal_mp : Outport
  AirCtl_bSmkDynLim : Outport  Port=2
  AirCtl_bSmkStatLim : Outport  Port=3
  wires:
  Delay/1 -> Switch2/3
  Switch3/1 -> Delay/1, AirCtl_rSmkCtlVal_mp/1  "AirCtl_rSmkCtlVal_mp"
  MinMax/1 -> Switch3/1
  Logical Operator/1 -> Switch3/2
  Switch1/1 -> Switch3/3
  Switch2/1 -> Switch1/3
  GetBit2/1(y) -> AirCtl_bSmkStatLim/1, Switch1/2, Logical Operator/2  "AirCtl_bSmkStatLim"
  GetBit1/1(y) -> Switch2/2, AirCtl_bSmkDynLim/1, Logical Operator/1  "AirCtl_bSmkDynLim"
  AirCtl_stAirCtlBits/1 -> GetBit1/1(u), GetBit2/1(u)
  Constant2/1 -> GetBit2/2(bit)
  Constant1/1 -> GetBit1/2(bit)
  Add1/1 -> MinMax/2, Switch1/1  "AirCtl_rSmkStat_mp"
  Add2/1 -> Switch2/1, MinMax/1  "AirCtl_rSmkDyn_mp"
  Divide1/1 -> Add1/2  "AirCtl_rEngTempSmkStatCorVal_mp"
  AirCtl_rSmkStat_MAP/1 -> Add1/1
  AirCtl_facEngTempSmkStatCor_CUR/1 -> Divide1/2
  AirCtl_rEngTempSmkStatCor_MAP/1 -> Divide1/1
  Divide3/1 -> Add2/2  "AirCtl_rEngTempSmkDynCorVal_mp"
  AirCtl_rSmkDyn_MAP/1 -> Add2/1
  AirCtl_facEngTempSmkDynCor_CUR/1 -> Divide3/2
  AirCtl_rEngTempSmkDynCor_MAP/1 -> Divide3/1
  AirCtl_tEngCtlVal_mp/1 -> AirCtl_facEngTempSmkDynCor_CUR/1, AirCtl_facEngTempSmkStatCor_CUR/1
  InjCtl_qSetUnBal/1 -> AirCtl_rSmkDyn_MAP/1, AirCtl_rSmkStat_MAP/1, AirCtl_rEngTempSmkStatCor_MAP/1, AirCtl_rEngTempSmkDynCor_MAP/1
  Epm_nEng/1 -> AirCtl_rSmkDyn_MAP/2, AirCtl_rEngTempSmkStatCor_MAP/2, AirCtl_rSmkStat_MAP/2, AirCtl_rEngTempSmkDynCor_MAP/2

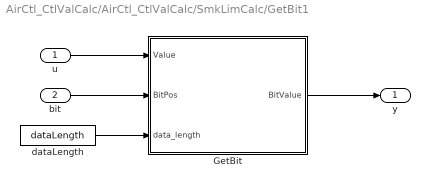
== system AirCtl_CtlValCalc/AirCtl_CtlValCalc/SmkLimCalc/GetBit1 ==
  u : Inport  OutDataTypeStr=uint32
  bit : Inport  Port=2
  GetBit : Stateflow chart  TreatAsAtomicUnit=on
  dataLength : Constant  Value=dataLength  OutDataTypeStr=uint8
  y : Outport  OutDataTypeStr=boolean
  wires:
  bit/1 -> GetBit/2(BitPos)
  u/1 -> GetBit/1(Value)
  GetBit/1(BitValue) -> y/1
  dataLength/1 -> GetBit/3(data_length)

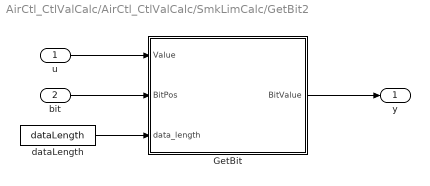
== system AirCtl_CtlValCalc/AirCtl_CtlValCalc/SmkLimCalc/GetBit2 ==
  u : Inport  OutDataTypeStr=uint32
  bit : Inport  Port=2
  GetBit : Stateflow chart  TreatAsAtomicUnit=on
  dataLength : Constant  Value=dataLength  OutDataTypeStr=uint8
  y : Outport  OutDataTypeStr=boolean
  wires:
  dataLength/1 -> GetBit/3(data_length)
  GetBit/1(BitValue) -> y/1
  u/1 -> GetBit/1(Value)
  bit/1 -> GetBit/2(BitPos)

== stateflow chart AirCtl_CtlValCalc/SmkLimCalc/GetBit1/GetBit ==
  (default) -> (junction 2)
  (junction 2) -> (junction 1) [order 1] : [BitPos < data_length]
  (junction 2) -> (junction 8) [order 2] : {BitValue = 0;}
  (junction 1) -> (junction 3) : {BitValue = (Value>>BitPos)&1;}
  (junction 3) -> (junction 8)
  (junction 8) -> (junction 6)
  data: Value input; BitPos input uint8; data_length input uint8; BitValue output boolean

== stateflow chart AirCtl_CtlValCalc/SmkLimCalc/GetBit2/GetBit ==
  (default) -> (junction 2)
  (junction 2) -> (junction 1) [order 1] : [BitPos < data_length]
  (junction 2) -> (junction 8) [order 2] : {BitValue = 0;}
  (junction 1) -> (junction 3) : {BitValue = (Value>>BitPos)&1;}
  (junction 3) -> (junction 8)
  (junction 8) -> (junction 6)
  data: Value input; BitPos input uint8; data_length input uint8; BitValue output boolean
